simulink model "simulink_ejemplo"  (R2016b)
settings: Solver=VariableStepAuto  StartTime=0.0  StopTime=10.0  RelTol=1e-3
settings Model: Creator=HP  LastModifiedBy=HP

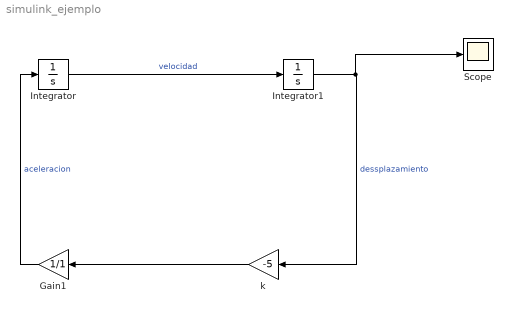
== system simulink_ejemplo ==
  Gain1 : Gain  Gain=1/1
  Integrator : Integrator
  Integrator1 : Integrator  InitialCondition=0.5
  Scope : Scope
  k : Gain  Gain=-5
  wires:
  Integrator/1 -> Integrator1/1  "velocidad"
  Integrator1/1 -> Scope/1, k/1  "dessplazamiento"
  k/1 -> Gain1/1
  Gain1/1 -> Integrator/1  "aceleracion"
